simulink model "IRB140"  (R2016b)
settings: Solver=ode113  StartTime=0.0  StopTime=40  RelTol=1e-3
(part 1 of 9)
settings Model: Creator=Roozbeh  LastModifiedBy=Roozbeh

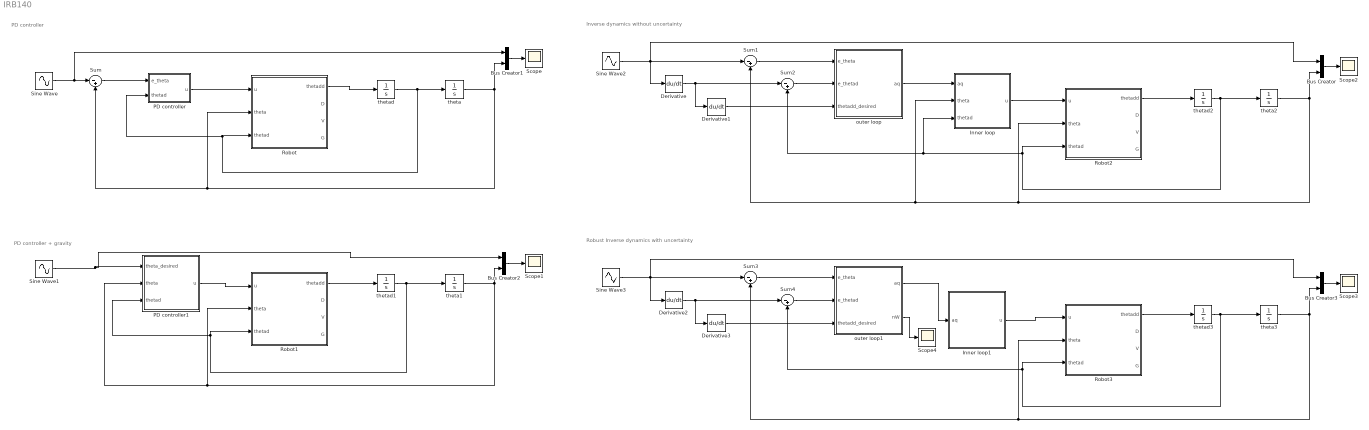
== system IRB140 ==
  note: PD controller + gravity
  note: PD controller
  note: Inverse dynamics without uncertainty
  note: Robust Inverse dynamics with uncertainty
  Bus Creator{,1..3} (4 alike) : BusCreator  Inputs=2
  Derivative{,1..3} (4 alike) : Derivative
  Inner loop : MATLAB Function  TreatAsAtomicUnit=on
  Inner loop1 : MATLAB Function  TreatAsAtomicUnit=on
  PD controller : MATLAB Function  TreatAsAtomicUnit=on
  PD controller1 : MATLAB Function  TreatAsAtomicUnit=on
  Robot : MATLAB Function  TreatAsAtomicUnit=on
  Robot1 : MATLAB Function  TreatAsAtomicUnit=on
  Robot2 : MATLAB Function  TreatAsAtomicUnit=on
  Robot3 : MATLAB Function  TreatAsAtomicUnit=on
  Scope{,1..4} (5 alike) : Scope
  Sine Wave : Sin  Amplitude=ones(6,1)  Bias=ones(6,1)  SampleTime=0
  Sine Wave1 : Sin  Amplitude=ones(6,1)  Bias=ones(6,1)  SampleTime=0
  Sine Wave2 : Sin  Amplitude=ones(6,1)  Bias=ones(6,1)  Frequency=0.1  SampleTime=0
  Sine Wave3 : Sin  Amplitude=ones(6,1)*0  Bias=ones(6,1)  Frequency=0.1  SampleTime=0
  Sum{,1..4} (5 alike) : Sum  Inputs=|-+
  outer loop : MATLAB Function  TreatAsAtomicUnit=on
  outer loop1 : MATLAB Function  TreatAsAtomicUnit=on
  theta{,1..3} (4 alike) : Integrator  InitialCondition=zeros(6,1)
  thetad{,1..3} (4 alike) : Integrator  InitialCondition=zeros(6,1)
  wires:
  thetad/1 -> PD controller/2(thetad), Robot/3(thetad), theta/1
  theta/1 -> Bus Creator1/2, Sum/2, Robot/2(theta)
  Robot/1(thetadd) -> thetad/1
  PD controller/1(u) -> Robot/1(u)
  Sum/1 -> PD controller/1(e_theta)
  thetad1/1 -> Robot1/3(thetad), PD controller1/3(thetad), theta1/1
  theta1/1 -> Bus Creator2/2, PD controller1/2(theta), Robot1/2(theta)
  Robot1/1(thetadd) -> thetad1/1
  PD controller1/1(u) -> Robot1/1(u)
  thetad2/1 -> Sum2/2, Inner loop/3(thetad), Robot2/3(thetad), theta2/1
  theta2/1 -> Bus Creator/2, Robot2/2(theta), Sum1/2, Inner loop/2(theta)
  Robot2/1(thetadd) -> thetad2/1
  Inner loop/1(u) -> Robot2/1(u)
  outer loop/1(aq) -> Inner loop/1(aq)
  Sum1/1 -> outer loop/1(e_theta)
  Sum2/1 -> outer loop/2(e_thetad)
  Derivative/1 -> Derivative1/1, Sum2/1
  Derivative1/1 -> outer loop/3(thetadd_desired)
  Sine Wave2/1 -> Bus Creator/1, Derivative/1, Sum1/1
  Sine Wave/1 -> Bus Creator1/1, Sum/1
  Sine Wave1/1 -> Bus Creator2/1, PD controller1/1(theta_desired)
  Bus Creator/1 -> Scope2/1
  Bus Creator1/1 -> Scope/1
  Bus Creator2/1 -> Scope1/1
  thetad3/1 -> theta3/1, Robot3/3(thetad), Sum4/2
  theta3/1 -> Sum3/2, Robot3/2(theta), Bus Creator3/2
  Robot3/1(thetadd) -> thetad3/1
  Inner loop1/1(u) -> Robot3/1(u)
  outer loop1/1(aq) -> Inner loop1/1(aq)
  Sum3/1 -> outer loop1/1(e_theta)
  Sum4/1 -> outer loop1/2(e_thetad)
  Derivative2/1 -> Sum4/1, Derivative3/1
  Derivative3/1 -> outer loop1/3(thetadd_desired)
  Sine Wave3/1 -> Sum3/1, Derivative2/1, Bus Creator3/1
  Bus Creator3/1 -> Scope3/1
  outer loop1/2(nW) -> Scope4/1

== matlab function IRB140/PD controller ==
  data: e_theta input; u output; thetad input
function u = fcn(e_theta, thetad)
Kp = diag([0.5 10 1 1 1 1])*100;
Kd = eye(6) * 10;
u = -Kp*e_theta - Kd*thetad;
